simulink model "SIL_MLX90316_Pedal"  (R2025b)
settings: Solver=FixedStepAuto  StartTime=0.0  StopTime=10.0  FixedStep=0.001  RelTol=1e-3  EnableMultiTasking=on
settings Model: ExtModeTrigDuration=2  Creator=Vinic  LastModifiedBy=Vinic
settings SolverCC: AutoInsertRateTranBlk=on
settings OptimizationCC: EnhancedBackFolding=on  PassReuseOutputArgsAs=Individual arguments  ZeroExternalMemoryAtStartup=off  ZeroInternalMemoryAtStartup=off  MaxStackSize=64  OptimizeBlockOrder=speed  DifferentSizesBufferReuse=on  OptimizationCustomize=off  EfficientTunableParamExpr=on
settings DebuggingCC: ParameterTunabilityLossMsg=error
settings HardwareCC: ProdBitPerInt=16.0  ProdBitPerPointer=16.0  ProdBitPerSizeT=16.0  ProdBitPerPtrDiffT=16.0  ProdLargestAtomicFloat=None  ProdWordSize=8.0  ProdHWDeviceType=Atmel->AVR
settings SFSimCC: MATLABDynamicMemAlloc=off
settings RTWCC: SystemTargetFile=ert.tlc  HardwareBoard=Arduino Leonardo  TemplateMakefile=ert_default_tmf  Toolchain=Arduino AVR  BuildConfiguration=Faster Runs  Description=Embedded Coder
settings CodeAppCC: ForceParamTrailComments=on  IgnoreCustomStorageClasses=off  OperatorAnnotations=on  SimulinkDataObjDesc=on  SFDataObjDesc=on  InsertBlockDesc=on
settings ERTTargetCC: ExtModeTransport=3.0  ExtModeStaticAlloc=on  ExtModeAutomaticAllocSize=off  ExtModeStaticAllocSize=250.0  ExtModeMexFile=ext_xcp  ExtModeIntrfLevel=Level2 - Open  InlinedParameterPlacement=Hierarchical  SupportContinuousTime=on  SupportVariableSizeSignals=on

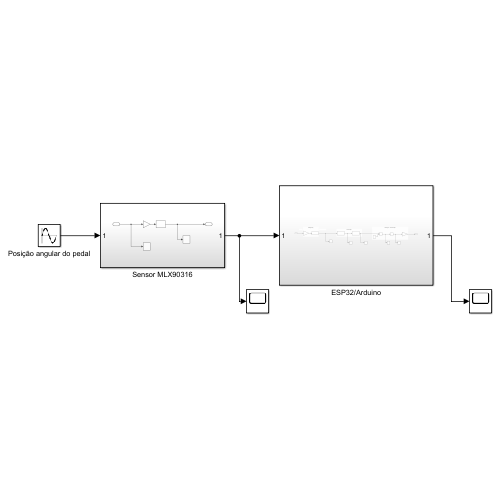
[thumbnail: Simulink's stored preview of the top-level diagram]
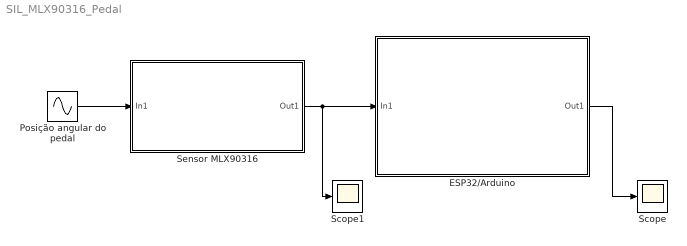
== system SIL_MLX90316_Pedal ==
  ESP32/Arduino : Subsystem
  Posição angular do pedal : Sin  Amplitude=20  Bias=50  Frequency=1.26  Phase=-1.57  SampleTime=0
  Scope : Scope
      settings: ActiveDisplayYMinimum=-12.484737484737481  ActiveDisplayYMaximum=112.36263736263736  DataLoggingVariableName=ScopeData7
  Scope1 : Scope
      settings: ActiveDisplayYMinimum=1.9345486657051936E-8  ActiveDisplayYMaximum=4.99999983428925  DataLoggingVariableName=ScopeData8
  Sensor MLX90316 : Subsystem
  wires:
  Sensor MLX90316/1(Out1) -> Scope1/1, ESP32/Arduino/1(In1)
  ESP32/Arduino/1(Out1) -> Scope/1
  Posição angular do pedal/1 -> Sensor MLX90316/1(In1)

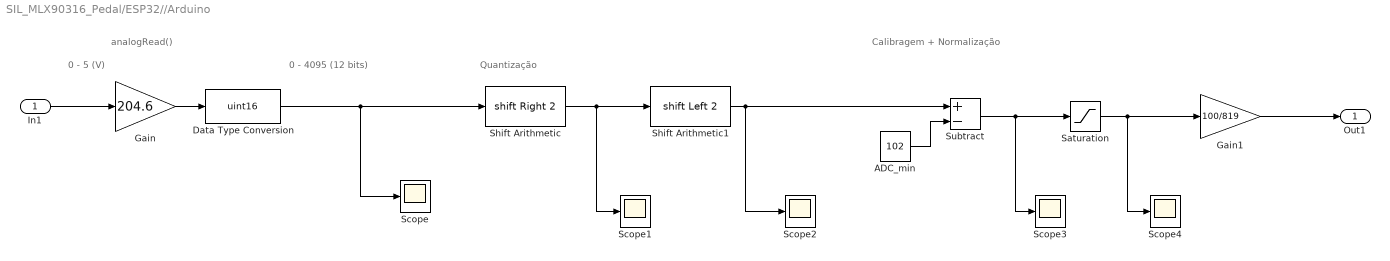
== system SIL_MLX90316_Pedal/ESP32//Arduino ==
  note: Calibragem + Normalização
  note: Quantização
  note: 0 - 5 (V)
  note: analogRead()
  note: 0 - 4095 (12 bits)
  In1 : Inport
  ADC_min : Constant  Value=102
  Data Type Conversion : DataTypeConversion  OutDataTypeStr=uint16  SaturateOnIntegerOverflow=off  RndMeth=Floor
  Gain : Gain  Gain=204.6
  Gain1 : Gain  Gain=100/819
  Saturation : Saturate  UpperLimit=819  LowerLimit=0
  Scope{,1..4} (5 alike) : Scope
      Scope settings: ActiveDisplayYMinimum=891.02605562551742  ActiveDisplayYMaximum=921.50737656283377  DataLoggingVariableName=ScopeData2
      Scope1 settings: ActiveDisplayYMinimum=-0.62499999999999289  ActiveDisplayYMaximum=255.625  DataLoggingVariableName=ScopeData3
      Scope2 settings: ActiveDisplayYMinimum=-2.4999999999999716  ActiveDisplayYMaximum=1022.5  DataLoggingVariableName=ScopeData4
      Scope3 settings: ActiveDisplayYMinimum=-9.5366057803248943  ActiveDisplayYMaximum=42.724262638871785  DataLoggingVariableName=ScopeData5
      Scope4 settings: ActiveDisplayYMinimum=-10.105449239040063  ActiveDisplayYMaximum=39.545410652833247  DataLoggingVariableName=ScopeData6
  Shift Arithmetic : ArithShift  BitShiftNumber=2  BitShiftDirection=Right
  Shift Arithmetic1 : ArithShift  BitShiftNumber=2  BitShiftDirection=Left
  Subtract : Sum  Inputs=+-
  Out1 : Outport
  wires:
  Gain1/1 -> Out1/1
  Gain/1 -> Data Type Conversion/1
  In1/1 -> Gain/1
  Data Type Conversion/1 -> Scope/1, Shift Arithmetic/1
  Shift Arithmetic/1 -> Scope1/1, Shift Arithmetic1/1
  Shift Arithmetic1/1 -> Subtract/1, Scope2/1
  ADC_min/1 -> Subtract/2
  Subtract/1 -> Saturation/1, Scope3/1
  Saturation/1 -> Scope4/1, Gain1/1

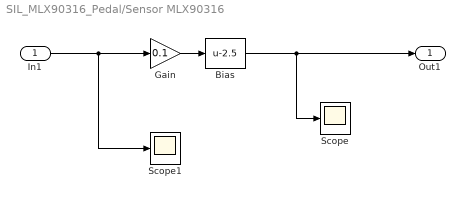
== system SIL_MLX90316_Pedal/Sensor MLX90316 ==
  In1 : Inport
  Bias : Bias  Bias=-2.5  SaturateOnIntegerOverflow=off
  Gain : Gain  Gain=0.1
  Scope : Scope
      settings: ActiveDisplayYMinimum=1.9345486657051936E-8  ActiveDisplayYMaximum=4.99999983428925
  Scope1 : Scope
      settings: ActiveDisplayYMinimum=25.000000193454866  ActiveDisplayYMaximum=74.9999983428925
  Out1 : Outport
  wires:
  In1/1 -> Scope1/1, Gain/1
  Gain/1 -> Bias/1
  Bias/1 -> Scope/1, Out1/1
